simulink model "Experiment_0121_840_161551_cs"  (R2019a)
settings: Solver=ode5  StartTime=0.0  StopTime=30  FixedStep=1/20  RelTol=1e-3
PreLoadFcn:
  | mbxruntime.callbacks.PreLoadFcn(bdroot);
PostLoadFcn:
  | mbxruntime.callbacks.PostLoadFcn(bdroot);
InitFcn:
  | mbxruntime.callbacks.InitFcn(bdroot);
StartFcn:
  | mbxruntime.callbacks.StartFcn(bdroot);
StopFcn:
  | mbxruntime.callbacks.StopFcn(bdroot);
model workspace (MAT data in the model file):
  mbox_table : struct (value not decoded)
  model_closed = 0
  sim_status = 0
undefined symbols (not defined in the file): DiscIntNeverNeededParam, warningInitialVelocity, x0
libraries: simulink x37, PreScanSimulinkLibrary x14, simulink_extras x10, PreScanUsefulBlocks x1
(part 6 of 6)

== system Experiment_0121_840_161551_cs/Ford_Focus_Stationwagon_1/Dynamics_Simple/Chassis/Bicycle_model_[XYZ]/X_Motion/Max RPM and zero- velocity detection/SR-Memory ==
  Signal : Inport
  Set : Inport  Port=2
  Reset : Inport  Port=3
  Constant : Constant  Value=0
  Detect Rise Positive : simulink/Logic and Bit Operations/Detect Rise Positive  vinit=0  InputProcessing=Inherited  OutDataTypeStr=uint8
  Detect Rise Positive1 : simulink/Logic and Bit Operations/Detect Rise Positive  vinit=0  InputProcessing=Inherited  OutDataTypeStr=uint8
  Manual Switch : ManualSwitch
  Manual Switch1 : ManualSwitch
  Switch : Switch  Criteria=u2 ~= 0
  Switch1 : Switch  Criteria=u2 ~= 0
  Unit Delay : UnitDelay  SampleTime=-1  HasFrameUpgradeWarning=on
  Out : Outport
  wires:
  Constant/1 -> Switch1/1
  Switch/1 -> Switch1/3
  Switch1/1 -> Unit Delay/1, Out/1
  Manual Switch1/1 -> Switch1/2
  Reset/1 -> Manual Switch1/2, Detect Rise Positive1/1
  Detect Rise Positive1/1 -> Manual Switch1/1
  Signal/1 -> Switch/1
  Unit Delay/1 -> Switch/3
  Set/1 -> Detect Rise Positive/1, Manual Switch/2
  Detect Rise Positive/1 -> Manual Switch/1
  Manual Switch/1 -> Switch/2

== matlab function Experiment_0121_840_161551_cs/Ford_Focus_Stationwagon_1/PathFollower_Preview_1/LateralController/CTRL REFERENCES/Calculate Lateral Error/eml_find_10k_lateral_error_points ==
  data: pvp input size=2; dist_psvehicle output size=10; TrajOffset_x_y_Y input size=3; ActorOffset_Left_Right input; p0 input size=2; PreviewDistance input size=10; Traj_x parameter; Traj_y parameter; Traj_t parameter; Traj_v parameter; RefreshCounter parameter
function dist_psvehicle  = eml_find_10k_lateral_error_points(pvp,TrajOffset_x_y_Y,ActorOffset_Left_Right,p0,PreviewDistance,Traj_x,Traj_y,Traj_t,Traj_v,RefreshCounter)

dist_psvehicle = emlfcn_find_10k_lateral_error_points(pvp,TrajOffset_x_y_Y,ActorOffset_Left_Right,p0,PreviewDistance,Traj_x,Traj_y,Traj_t,Traj_v,RefreshCounter);

% end function

== stateflow chart Experiment_0121_840_161551_cs/Ford_Focus_Stationwagon_1/Subsystem/Chart ==
  state failure
    en,du:
    fcw_flag=0;
  state on
    state has_target
      state nowarning
        en,du:
        fcw_flag=0;
        enable =fcw_enable(1);
      state warning
        en,du:
        fcw_flag=1;
        enable =fcw_enable(1);
      (default) -> nowarning
      nowarning -> warning : [TTC(1)<2.3]
      warning -> nowarning : after(4,sec)
    state no_target
      en,du:
      fcw_flag=0;
      enable =fcw_enable(1);
    (default) -> no_target
    no_target -> has_target : [fcw_enable(1)>0]
    has_target -> no_target : [0]
  state off
    en,du:
    fcw_flag=0
  on -> failure [order 2] : [0]
  (default) -> off
  off -> on : [switchon==1]
  on -> off [order 1] : [switchon==0]
  data: fcw_flag output; switchon input; fcw_enable input; TTC input; ETTC input; fail input; enable output

== matlab function Experiment_0121_840_161551_cs/Ford_Focus_Stationwagon_1/PathFollower_Preview_1/LateralController/CTRL REFERENCES/Find Reference Point (pref0) on Trajectory closest to P0 Point (p0)/eml_find_closest_trajectory_points0 ==
  data: pvp input size=2; Actor_traj_distance output; TrajOffset_x_y_Y input size=3; ActorOffset_Left_Right input; p0 input size=3; Traj_x parameter; Traj_y parameter; Actor_traj_angle output; RefreshCounter parameter
function [Actor_traj_distance,Actor_traj_angle]  = eml_find_closest_trajectory_points0(pvp,TrajOffset_x_y_Y,ActorOffset_Left_Right,p0,Traj_x,Traj_y,RefreshCounter)

[Actor_traj_distance,Actor_traj_angle]  = emlfcn_find_closest_trajectory_points0(pvp,TrajOffset_x_y_Y,ActorOffset_Left_Right,p0,Traj_x,Traj_y,RefreshCounter);

% end function

== matlab function Experiment_0121_840_161551_cs/Ford_Focus_Stationwagon_1/PathFollower_Preview_1/LateralController/Calculate delta steering error/eml_delta_steering_error ==
  data: v_x_vehicle input; v_x_vehicle_Min input; t_Preview_LatCtrl input; delta_steeringwheeltotal output; v_y_vehicle input; yawrate_vehicle input; CorneringStiffness_Tyres_Front input; CorneringStiffness_Tyres_Rear input; m_vehicle_total input; inertia_z_vehicle_total input; e_Lat input size=10; Pos_x_CoG_Vehicle input; wheelbase input; RefreshCounter parameter
function delta_steeringwheeltotal = eml_delta_steering_error(v_x_vehicle,v_x_vehicle_Min,t_Preview_LatCtrl,v_y_vehicle,yawrate_vehicle,CorneringStiffness_Tyres_Front,CorneringStiffness_Tyres_Rear,m_vehicle_total,inertia_z_vehicle_total,e_Lat,Pos_x_CoG_Vehicle,wheelbase,RefreshCounter)

delta_steeringwheeltotal = emlfcn_delta_steering_error(v_x_vehicle,v_x_vehicle_Min,t_Preview_LatCtrl,v_y_vehicle,yawrate_vehicle,CorneringStiffness_Tyres_Front,CorneringStiffness_Tyres_Rear,m_vehicle_total,inertia_z_vehicle_total,e_Lat,Pos_x_CoG_Vehicle,wheelbase,RefreshCounter);

% end function
